simulink model "modelling_of_electrical_power_system"  (R2019a)
settings: Solver=VariableStepAuto  StartTime=0.0  StopTime=0.5  RelTol=1e-3
undefined symbols (not defined in the file): D1, Delta
libraries: powerlib x10
settings Model: Creator=Soham Kundu  LastModifiedBy=Soham Kundu

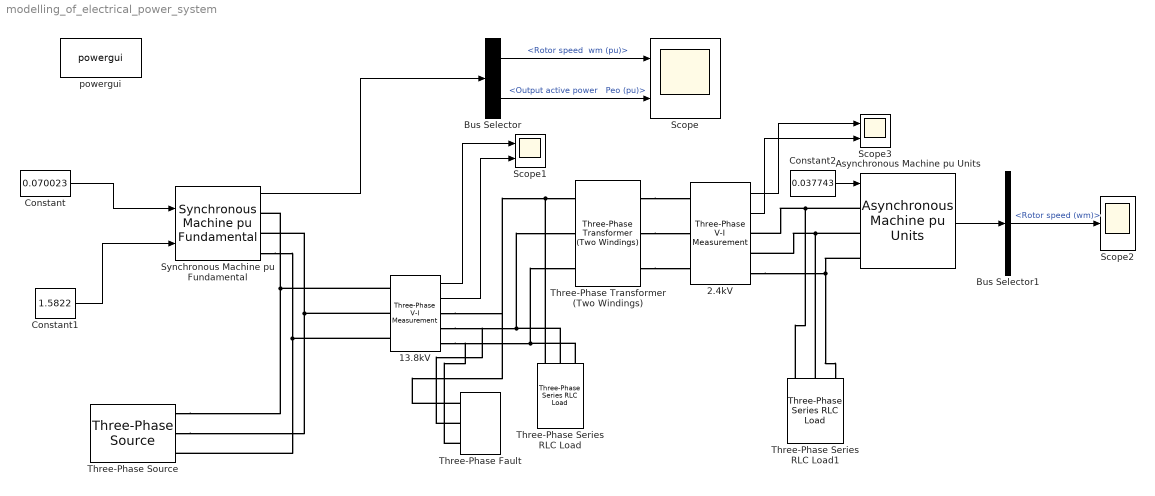
== system modelling_of_electrical_power_system ==
  13.8kV : powerlib/Measurements/Three-Phase V-I Measurement  VoltageMeasurement=phase-to-ground  SetLabelV=off  LabelV=Vabc  Vpu=off  VpuLL=off  CurrentMeasurement=yes  SetLabelI=off  LabelI=Iabc  Ipu=off  Pbase=100e6  Vbase=500e3  OutputType=Complex  PhasorSimulation=off  PSBequivalent=0
      settings: SourceProductName=Simscape Electrical
  2.4kV : powerlib/Measurements/Three-Phase V-I Measurement  VoltageMeasurement=phase-to-ground  SetLabelV=off  LabelV=Vabc  Vpu=off  VpuLL=off  CurrentMeasurement=yes  SetLabelI=off  LabelI=Iabc  Ipu=off  Pbase=100e6  Vbase=500e3  OutputType=Complex  PhasorSimulation=off  PSBequivalent=0
      settings: SourceProductName=Simscape Electrical
  Asynchronous Machine pu Units : powerlib/Machines/Asynchronous Machine pu Units  RotorType=Squirrel-cage  PresetModel=No  MechanicalLoad=Torque Tm  ShowDetailedParameters=on  ReferenceFrame=Rotor  Units=pu  MeasurementBus=off  NominalParameters=[1.6e+05 400 50]  Stator=[0.01379 0.04775]  Rotor=[0.007728 0.04775]  Cage1=[0.01909 0.0397]  Cage2=[0.01909 0.0397]  Lm=2.416  Mechanical=[0.2236 0.008726 2]  PolePairs=2  InitialConditions=[0.172021 0 120.657 120.657 120.657 -103.79 -223.79 16.2105]  SimulateSaturation=off  Saturation="[0.212,0.4201,0.8125,1.0979,1.4799,2.2457,3.2586,4.5763,6.4763 ;   0.5,0.7,0.9,1,1.1,1.2 ,1.3,1.4,1.5]"  LoadFlowParameters=0  TsPowergui=0  TsBlock=-1  IterativeModel=Trapezoidal non iterative  IterativeDiscreteModel=Trapezoidal non iterative  Pmec=5000
      settings: SourceProductName=Simscape Electrical  SourceProductBaseCode=PS
  Bus Selector : BusSelector  OutputSignals="Mechanical.Rotor speed  wm (pu),Output active power   Peo (pu)"
  Bus Selector1 : BusSelector  OutputSignals=Mechanical.Rotor speed (wm)
  Constant : Constant  Value=0.070023
  Constant1 : Constant  Value=1.5822
  Constant2 : Constant  Value=0.037743
  Scope : Scope  NumInputPorts=2
  Scope1 : Scope  NumInputPorts=2
  Scope2 : Scope
  Scope3 : Scope  NumInputPorts=2
  Synchronous Machine pu Fundamental : powerlib/Machines/Synchronous Machine pu Fundamental  PresetModel=No  MechanicalLoad=Mechanical power Pm  ShowDetailedParameters=on  RotorType=Salient-pole  Units=per unit fundamental parameters  MeasurementBus=off  NominalParameters="[ 250E6  13800   50]"  Stator="[ 2.85E-03  0.114  1.19  0.36 ]"  Field="[ 5.79E-04  0.114]"  Dampers2=[0.0652, 0.5134, 0.0287, 0.2553, 7.765e-3, 0.9167 ]  Dampers1="[ 1.17E-02  0.182  1.97E-02  0.384 ]"  Mechanical=[ 3.7 0 20]  PolePairs=20  InitialConditions=[0 -88.5031 0.450324 0.450324 0.450324 -81.129 -201.129 38.871 1.58219]  SetSaturation=off  Saturation=[0.6404,0.7127,0.8441,0.9214,0.9956,1.082,1.19,1.316,1.457;0.7,0.7698,0.8872,0.9466,0.9969,1.046,1.1,1.151,1.201]  LoadFlowParameters=[1,0,0,0,0]  TsPowergui=0  TsBlock=-1  IterativeModel=Trapezoidal non iterative  IterativeDiscreteModel=Trapezoidal non iterative  BusType=PV  Pref=250e6  Qref=0  Qmin=-inf  Qmax=inf  PLF=0  QLF=0
      settings: SourceProductName=Simscape Electrical  SourceProductBaseCode=PS
  Three-Phase Series RLC Load : powerlib/Elements/Three-Phase Series RLC Load  LConnTagsString=A|B|C  Configuration=Y (grounded)  NominalVoltage=(13800)*1  Vabc=[1e3 1e3 1e3]  Vabcp=[1e3 1e3 1e3]  NominalFrequency=50  UnbalancedPower=off  ActivePower=10e3  InductivePower=10e3  CapacitivePower=10e3  Pabc=[10e3 9e3 11e3]  QLabc=[100 90 110]  QCabc=[100 90 110]  Pabcp=[10e3 9e3 11e3]  QLabcp=[100 90 110]  QCabcp=[100 90 110]  Measurements=None  LoadType=constant PQ
      settings: SourceProductName=Simscape Electrical
  Three-Phase Series RLC Load1 : powerlib/Elements/Three-Phase Series RLC Load  LConnTagsString=A|B|C  Configuration=Y (grounded)  NominalVoltage=(400)*5.9969  Vabc=[1e3 1e3 1e3]  Vabcp=[1e3 1e3 1e3]  NominalFrequency=50  UnbalancedPower=off  ActivePower=10e3  InductivePower=10e3  CapacitivePower=0  Pabc=[10e3 9e3 11e3]  QLabc=[100 90 110]  QCabc=[100 90 110]  Pabcp=[10e3 9e3 11e3]  QLabcp=[100 90 110]  QCabcp=[100 90 110]  Measurements=None  LoadType=constant PQ
      settings: SourceProductName=Simscape Electrical
  Three-Phase Transformer (Two Windings) : powerlib/Elements/Three-Phase Transformer (Two Windings)  Winding1Connection=Yg  Winding2Connection=Delta (D1)  CoreType=Three single-phase transformers  SetSaturation=off  Hysteresis=off  DataFile='hysteresis'  SetInitialFlux=off  Measurements=None  UNITS=pu  NominalPower=[ 250e6 , 50 ]  Winding1=[13.8e+03 0.002 0]  Winding2=[2400 0.002 0]  Rm=Inf  Lm=Inf  L0=2.866  Saturation=[0 0;0.0024 1.2;1 1.52]  InitialFluxes=[1273.5 -1273.5 1114.3]  BreakLoop=off  DiscreteSolver=Trapezoidal iterative  DataType=off  TransfoNumber=1
      settings: SourceProductName=Simscape Electrical
  Three-Phase Fault : powerlib/Elements/Three-Phase Fault  InitialStates=0  FaultA=on  FaultB=on  FaultC=on  GroundFault=on  SwitchTimes="[1/50  3/50]"  External=off  SwitchStatus=NaN  FaultResistance=0.001  GroundResistance=0.01  SnubberResistance=1e6  SnubberCapacitance=inf  Measurements=Fault voltages and currents
      settings: SourceProductName=Simscape Electrical
  Three-Phase Source : powerlib/Electrical Sources/Three-Phase Source  InternalConnection=Yg  VoltagePhases=off  Voltage=(13800)*1.14627  PhaseAngle=20.9723  Voltage_phases=[25e3 25e3 25e3]/sqrt(3)  PhaseAngles_phases=[0 -120 +120]  Frequency=50  NonIdealSource=on  SpecifyImpedance=off  Resistance=0.8929  Inductance=16.58e-3  ShortCircuitLevel=100e6  BaseVoltage=25e3  XRratio=7  BusType=swing  Pref=15e6  Qref=0  Prefabc=[10e3, 10e3, 10e3]  Qrefabc=[0, 0, 0]  Qmin=-inf  Qmax=inf
      settings: SourceProductName=Simscape Electrical
  powergui : powerlib/powergui  Priority=1  SimulationMode=Continuous  SampleTime=50e-6  frequency=60  Iterations=50  frequencyindice=50  Pbase=100e6  ErrMax=0.0001  UnitsV=kV  UnitsW=MW  buscounter=0  FunctionMessages=off  echomessages=off  EnableUseOfTLC=off  CurrentSourceSwitches=off  DisableSnubberDevices=off  DisableRonSwitches=off  DisableVfSwitches=off  DisplayEquations=off  AutomaticDiscreteSolvers=off  SolverType=Tustin/Backward Euler (TBE)  Interpol=off  ExternalGateDelay=off  methode=off  Ts=100  x0status=blocks  SPID=on  SwTol=0  HookPort=off  NonlinearTolerance=0  nMaxIteration=15  ContinueOnMaxIteration=off  RestoreLinks=warning  ResistiveCurrentMeasurement=off  Frange=[0:2:500]  Ylog=off  Xlog=on  ShowGrid=off  save=off  variable=ZData  structure=0  ZoomFFT=off  StartTime=0.0  cycles=1  DisplayStyle=1  fundamental=60  FreqAxis=off  MaxFrequency=1000  frequencyindicesteady=1  RmsSteady=1  display=off
      settings: SourceProductName=Simscape Electrical
  wires:
  Constant/1 -> Synchronous Machine pu Fundamental/1
  Bus Selector/1 -> Scope/1  "<Rotor speed  wm (pu)>"
  Bus Selector/2 -> Scope/2  "<Output active power   Peo (pu)>"
  Constant1/1 -> Synchronous Machine pu Fundamental/2
  Synchronous Machine pu Fundamental/1 -> Bus Selector/1
  Constant2/1 -> Asynchronous Machine pu Units/1
  13.8kV/1 -> Scope1/1
  13.8kV/2 -> Scope1/2
  Asynchronous Machine pu Units/1 -> Bus Selector1/1
  Bus Selector1/1 -> Scope2/1  "<Rotor speed (wm)>"
  2.4kV/1 -> Scope3/1
  2.4kV/2 -> Scope3/2
  connections:
  Three-Phase Series RLC Load/LConn1 -- 13.8kV/RConn1 -- Three-Phase Fault/LConn1 -- Three-Phase Transformer (Two Windings)/LConn1
  Three-Phase Series RLC Load/LConn2 -- 13.8kV/RConn2 -- Three-Phase Fault/LConn2 -- Three-Phase Transformer (Two Windings)/LConn2
  Three-Phase Series RLC Load/LConn3 -- 13.8kV/RConn3 -- Three-Phase Fault/LConn3 -- Three-Phase Transformer (Two Windings)/LConn3
  Asynchronous Machine pu Units/LConn1 -- Three-Phase Series RLC Load1/LConn1 -- 2.4kV/RConn1
  Asynchronous Machine pu Units/LConn2 -- Three-Phase Series RLC Load1/LConn2 -- 2.4kV/RConn2
  Asynchronous Machine pu Units/LConn3 -- 2.4kV/RConn3 -- Three-Phase Series RLC Load1/LConn3
  Three-Phase Transformer (Two Windings)/RConn1 -- 2.4kV/LConn1
  Three-Phase Transformer (Two Windings)/RConn2 -- 2.4kV/LConn2
  Three-Phase Transformer (Two Windings)/RConn3 -- 2.4kV/LConn3
  Three-Phase Source/RConn1 -- 13.8kV/LConn1 -- Synchronous Machine pu Fundamental/RConn1
  Three-Phase Source/RConn2 -- 13.8kV/LConn2 -- Synchronous Machine pu Fundamental/RConn2
  Synchronous Machine pu Fundamental/RConn3 -- 13.8kV/LConn3 -- Three-Phase Source/RConn3
